simulink model "transferfunction9B"  (R2022b)
settings: Solver=VariableStepAuto  StartTime=0  StopTime=t(end)  FixedStep=t(2)-t(1)  MaxStep=Auto  MinStep=Auto  RelTol=1e-3
values from neighbouring files (symbols this model uses):
  Kc = 0.25    [transferfunction9_Kobe_Michiels.m]
settings Model: Creator=u0062516  LastModifiedBy=Kobe Michiels
settings SolverCC: InitialStep=Auto
settings DataIOCC: ExternalInput=[t input]  LoadExternalInput=on  SaveFormat=Array  SignalLogging=off  DSMLogging=off  OutputSaveName=y  ReturnWorkspaceOutputsName=tpaa9b6cbf_e618_439f_8d7a_ff7f543ec0c7
settings HardwareCC: TargetBitPerPointer=64  TargetBitPerSizeT=64  TargetBitPerPtrDiffT=64  TargetLongLongMode=on  TargetIntDivRoundTo=Zero  TargetEndianess=LittleEndian  TargetWordSize=64  TargetHWDeviceType=MATLAB Host  ProdEqTarget=off
settings RTWCC: Description=Rapid Simulation Target  SystemTargetFile=rsim.tlc  TemplateMakefile=rsim_default_tmf
settings RSimTargetCC: TargetLangStandard=C99 (ISO)  OptimizeReductions=off

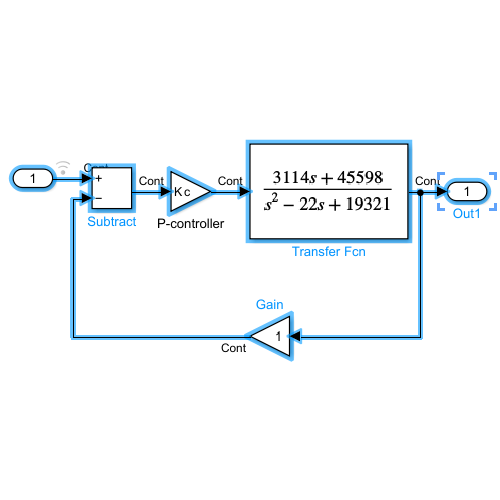
[thumbnail: Simulink's stored preview of the top-level diagram]
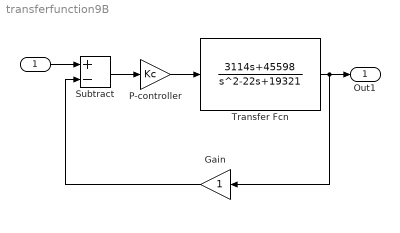
== system transferfunction9B ==
  " " : Inport
  Gain : Gain
  P-controller : Gain  Gain=Kc
  Subtract : Sum  Inputs=+-
  Transfer Fcn : TransferFcn  Numerator=[3114 45598]  Denominator=[1 -22 19321]  ParameterTunability=Unconstrained
  Out1 : Outport
  wires:
  Transfer Fcn/1 -> Gain/1, Out1/1
  Gain/1 -> Subtract/2
  Subtract/1 -> P-controller/1
  " "/1 -> Subtract/1
  P-controller/1 -> Transfer Fcn/1
